simulink model "mdl02_ctrlCompare"  (R2021a)
settings: Solver=FixedStepAuto  StartTime=0.0  StopTime=T  FixedStep=Ts  RelTol=1e-3
values from neighbouring files (symbols this model uses):
  intLim = 3    [Sim01_antiwindup.m]    (also in Sim02_ctrlCompare.m = 1)
  Ka = 500    [Sim01_antiwindup.m]    (also in Sim02_ctrlCompare.m = 50)
  Ki = 4    [Sim02_ctrlCompare.m]
  Kp = 2    [Sim02_ctrlCompare.m]
  stepAmp = [1, -1]    [Sim01_antiwindup.m]    (also in Sim02_ctrlCompare.m = [0 1])
  stepTime = 5    [Sim01_antiwindup.m]    (also in Sim02_ctrlCompare.m = 0)
settings Model: Creator=xiaocy  LastModifiedBy=xiaocy
settings DataIOCC: ReturnWorkspaceOutputs=off

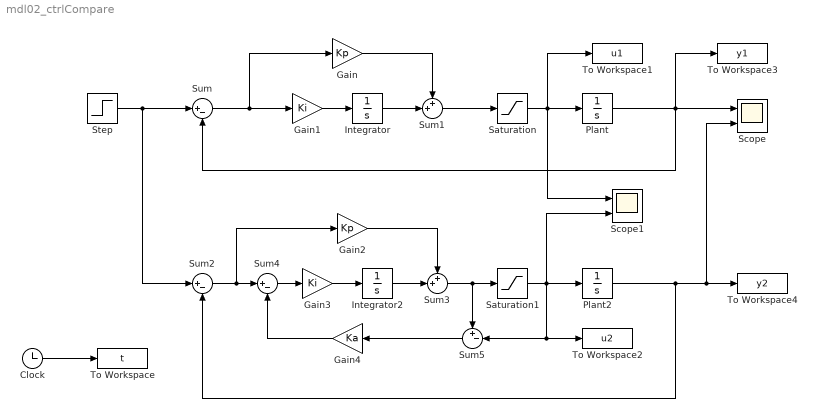
== system mdl02_ctrlCompare ==
  Clock : Clock
  Gain : Gain  Gain=Kp
  Gain1 : Gain  Gain=Ki
  Gain2 : Gain  Gain=Kp
  Gain3 : Gain  Gain=Ki
  Gain4 : Gain  Gain=Ka
  Integrator : Integrator
  Integrator2 : Integrator
  Plant : Integrator
  Plant2 : Integrator
  Saturation : Saturate  UpperLimit=intLim  LowerLimit=-intLim
  Saturation1 : Saturate  UpperLimit=intLim  LowerLimit=-intLim
  Scope : Scope  NumInputPorts=2
  Scope1 : Scope  NumInputPorts=2
  Step : Step  Time=stepTime  Before=stepAmp(1)  After=stepAmp(2)  SampleTime=0
  Sum : Sum  Inputs=|+-
  Sum1 : Sum  Inputs=++|
  Sum2 : Sum  Inputs=|+-
  Sum3 : Sum  Inputs=++|
  Sum4 : Sum  Inputs=|+-
  Sum5 : Sum  Inputs=+-|
  To Workspace : ToWorkspace  VariableName=t  SampleTime=-1
  To Workspace1 : ToWorkspace  VariableName=u1  SampleTime=-1
  To Workspace2 : ToWorkspace  VariableName=u2  SampleTime=-1
  To Workspace3 : ToWorkspace  VariableName=y1  SampleTime=-1
  To Workspace4 : ToWorkspace  VariableName=y2  SampleTime=-1
  wires:
  Clock/1 -> To Workspace/1
  Saturation/1 -> To Workspace1/1, Scope1/1, Plant/1
  Sum/1 -> Gain1/1, Gain/1
  Gain1/1 -> Integrator/1
  Integrator/1 -> Sum1/2
  Sum1/1 -> Saturation/1
  Gain/1 -> Sum1/1
  Plant/1 -> To Workspace3/1, Scope/1, Sum/2
  Plant2/1 -> Scope/2, To Workspace4/1, Sum2/2
  Gain2/1 -> Sum3/1
  Sum3/1 -> Saturation1/1, Sum5/1
  Integrator2/1 -> Sum3/2
  Gain3/1 -> Integrator2/1
  Sum2/1 -> Gain2/1, Sum4/1
  Saturation1/1 -> Scope1/2, Plant2/1, To Workspace2/1, Sum5/2
  Step/1 -> Sum2/1, Sum/1
  Sum4/1 -> Gain3/1
  Gain4/1 -> Sum4/2
  Sum5/1 -> Gain4/1
